simulink model "two_link_model_controller"  (R2020b)
settings: Solver=ode45  StartTime=0.0  StopTime=3  RelTol=1e-3  EnableMultiTasking=on
model workspace (MAT data in the model file):
  q_d_start = [0 0]
  q_d_stop = [1.57079632679 1.57079632679]
undefined symbols (not defined in the file or in its folder): F, K_D, K_P
settings Model: OrderedModelArguments=off  Creator=kma  LastModifiedBy=fridamei
settings DataIOCC: LimitDataPoints=on  SaveFormat=Array  ReturnWorkspaceOutputs=off
settings OptimizationCC: LifeSpan=inf
settings DebuggingCC: SFUnexpectedBacktrackingDiag=warning  SFNoUnconditionalDefaultTransitionDiag=warning  SFExecutionAtInitializationDiag=none  ArithmeticOperatorsInVariantConditions=warning
settings HardwareCC: ProdBitPerPointer=32  ProdBitPerSizeT=32  ProdBitPerPtrDiffT=32  ProdLargestAtomicFloat=None  ProdIntDivRoundTo=Undefined  ProdEndianess=Unspecified  ProdWordSize=32  ProdHWDeviceType=32-bit Generic
settings ModelReferenceCC: PropagateSignalLabelsOutOfModel=off
settings SFSimCC: SimUseLocalCustomCode=off  CustomCodeUndefinedFunction=UseInterfaceOnly
settings RTWCC: RTWUseLocalCustomCode=off
settings CodeAppCC: StateflowObjectComments=on
settings GRTTargetCC: TargetLangStandard=C89/C90 (ANSI)
settings ConfigComp: CovMetricSettings=dw  CovSaveCumulativeToWorkspaceVar=on  CovSaveSingleToWorkspaceVar=on  CovExternalEMLEnable=off

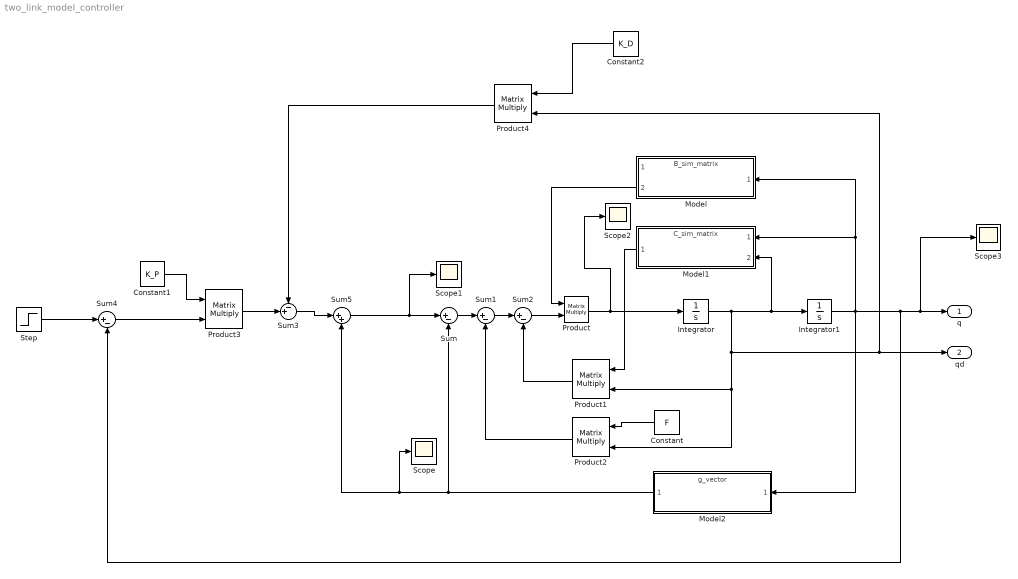
== system two_link_model_controller ==
  Constant : Constant  Value=F
  Constant1 : Constant  Value=K_P
  Constant2 : Constant  Value=K_D
  Integrator : Integrator
  Integrator1 : Integrator
  Model : ModelReference  ModelNameDialog=B_sim_matrix.slx  SimulationMode=Normal  ModelReferenceVersion=1.6
  Model1 : ModelReference  ModelNameDialog=C_sim_matrix.slx  SimulationMode=Normal  ModelReferenceVersion=1.2
  Model2 : ModelReference  ModelNameDialog=g_vector.slx  SimulationMode=Normal  ModelReferenceVersion=1.8
  Product{,1..4} (5 alike) : Product  Multiplication=Matrix(*)
  Scope{,1..3} (4 alike) : Scope
  Step : Step  Before=q_d_start  After=q_d_stop  SampleTime=0
  Sum{,1..2,4} (4 alike) : Sum  Inputs=|+-
  Sum3 : Sum  Inputs=-+|
  Sum5 : Sum  Inputs=|++
  q : Outport  PortDimensions=2
  qd : Outport  Port=2  PortDimensions=2
  wires:
  Product/1 -> Scope2/1, Integrator/1
  Model/2 -> Product/1
  Model1/1 -> Product1/1
  Constant/1 -> Product2/1
  Sum/1 -> Sum1/1
  Sum1/1 -> Sum2/1
  Sum2/1 -> Product/2
  Product1/1 -> Sum2/2
  Product2/1 -> Sum1/2
  Model2/1 -> Sum5/2, Scope/1, Sum/2
  Sum5/1 -> Scope1/1, Sum/1
  Integrator/1 -> Product4/2, qd/1, Product2/2, Product1/2, Model1/2, Integrator1/1
  Step/1 -> Sum4/1
  Sum4/1 -> Product3/2
  Constant1/1 -> Product3/1
  Product3/1 -> Sum3/2
  Sum3/1 -> Sum5/1
  Constant2/1 -> Product4/1
  Product4/1 -> Sum3/1
  Integrator1/1 -> Model2/1, Sum4/2, Scope3/1, q/1, Model/1, Model1/1
